simulink model "pfb_fft"  (Simulink 7.0)
settings: Solver=FixedStepDiscrete  SolverMode=SingleTasking  StartTime=0.0  StopTime=2500  RelTol=1e-3
libraries: xbsIndex_r4 x1144
(part 12 of 20)

== system pfb_fft/r4_dit_fft/r4_dit_stage_5/r4_butterfly/butterfly2 ==
  a : Inport  OutDataType=sfix(16)  OutScaling=2^0
  b : Inport  Port=2  OutDataType=sfix(16)  OutScaling=2^0
  sync_in : Inport  Port=3  OutDataType=sfix(16)  OutScaling=2^0
  Delay : xbsIndex_r4/Delay  en=off  latency=1  dbl_ovrd=off  reg_retiming=off  block_type=delay
      settings: xl_area=[1 1 0 0 0 0 0]
  add_im : xbsIndex_r4/AddSub  mode=Addition  use_carryin=off  use_carryout=off  en=off  latency=1  precision=Full  arith_type=Unsigned  n_bits=8  bin_pt=2  quantization=Truncate  overflow=Wrap  dbl_ovrd=off  use_behavioral_HDL=on  pipelined=on  use_rpm=on  hw_selection=Fabric  block_type=addsub
      settings: xl_area=[10 19 0 19 0 0 0]  block_version=10.1.3
  add_re : xbsIndex_r4/AddSub  mode=Addition  use_carryin=off  use_carryout=off  en=off  latency=1  precision=Full  arith_type=Unsigned  n_bits=8  bin_pt=2  quantization=Truncate  overflow=Wrap  dbl_ovrd=off  use_behavioral_HDL=on  pipelined=on  use_rpm=on  hw_selection=Fabric  block_type=addsub
      settings: xl_area=[10 19 0 19 0 0 0]  block_version=10.1.3
  c_to_ri : Subsystem  mask(Complex to Real-Imag){n_bits=18, bin_pt=0}
      mask prompts: n_bits "Bit Width"; bin_pt "Binary Point"
      mask help: Outputs real and imaginary components of a complex input.
      settings: AttributesFormatString=18_0 r/i
      mask Help:
      | <pre>
      | Description::
      | 
      | Outputs real and imaginary components of a complex input.
      | Useful for simplifying interconnects.
      | See also: Real-Imag to Complex (ri_to_c)
      | 
      | Mask Parameters::
      | 
      | Bit Width (n_bits): Specifies the width of the real/imaginary components.
      | Assumed equal for both components.
      | 
      | Binary Point (bin_pt): Specifies the binary point location in the real/imaginary components.
      | Assumed equal for both components.
      | </pre>
  c_to_ri1 : Subsystem  mask(Complex to Real-Imag){n_bits=18, bin_pt=0}
      mask prompts: n_bits "Bit Width"; bin_pt "Binary Point"
      mask help: Outputs real and imaginary components of a complex input.
      settings: AttributesFormatString=18_0 r/i
      mask Help:
      | <pre>
      | Description::
      | 
      | Outputs real and imaginary components of a complex input.
      | Useful for simplifying interconnects.
      | See also: Real-Imag to Complex (ri_to_c)
      | 
      | Mask Parameters::
      | 
      | Bit Width (n_bits): Specifies the width of the real/imaginary components.
      | Assumed equal for both components.
      | 
      | Binary Point (bin_pt): Specifies the binary point location in the real/imaginary components.
      | Assumed equal for both components.
      | </pre>
  requant{0..3} (4 alike) : xbsIndex_r4/Convert  arith_type="Signed  (2's comp)"  n_bits=19  bin_pt=0  quantization=Truncate  overflow=Wrap  latency=0  dbl_ovrd=off  pipeline=on  block_type=convert
      settings: xl_area=[0 0 0 0 0 0 0]  block_version=10.1.3
  ri_to_c : Subsystem
      mask Type: Real-Imag to Complex
      mask Description: Concatenates real and imaginary inputs into a complex output.
      mask Help:
      | <pre>
      | Description::
      | 
      | Concatenates a real and imaginary input into a complex output.
      | Useful for simplifying interconnects.
      | See also: Complex to Real-Imag (c_to_ri)
      | 
      | Mask Parameters::
      | 
      | (N/A)
      | </pre>
  ri_to_c1 : Subsystem
      mask Type: Real-Imag to Complex
      mask Description: Concatenates real and imaginary inputs into a complex output.
      mask Help:
      | <pre>
      | Description::
      | 
      | Concatenates a real and imaginary input into a complex output.
      | Useful for simplifying interconnects.
      | See also: Complex to Real-Imag (c_to_ri)
      | 
      | Mask Parameters::
      | 
      | (N/A)
      | </pre>
  shift{0..3} (4 alike) : xbsIndex_r4/Scale  scale_factor=0  dbl_ovrd=off  block_type=scale
      settings: infoedit=Scales input by a power of two by adjusting the binary point position.<P><P>Hardware notes: In hardware this block costs nothing.  block_version=10.1.3
  sub_im : xbsIndex_r4/AddSub  mode=Subtraction  use_carryin=off  use_carryout=off  en=off  latency=1  precision=Full  arith_type=Unsigned  n_bits=8  bin_pt=2  quantization=Truncate  overflow=Wrap  dbl_ovrd=off  use_behavioral_HDL=on  pipelined=on  use_rpm=on  hw_selection=Fabric  block_type=addsub
      settings: xl_area=[10 19 0 19 0 0 0]  block_version=10.1.3
  sub_re : xbsIndex_r4/AddSub  mode=Subtraction  use_carryin=off  use_carryout=off  en=off  latency=1  precision=Full  arith_type=Unsigned  n_bits=8  bin_pt=2  quantization=Truncate  overflow=Wrap  dbl_ovrd=off  use_behavioral_HDL=on  pipelined=on  use_rpm=on  hw_selection=Fabric  block_type=addsub
      settings: xl_area=[10 19 0 19 0 0 0]  block_version=10.1.3
  a+b : Outport  OutDataType=sfix(16)  OutScaling=2^0
  a-b : Outport  Port=2  OutDataType=sfix(16)  OutScaling=2^0
  sync_out : Outport  Port=3  OutDataType=sfix(16)  OutScaling=2^0
  wires:
  shift3/1 -> requant3/1
  sub_im/1 -> shift3/1
  shift2/1 -> requant2/1
  sub_re/1 -> shift2/1
  shift1/1 -> requant1/1
  shift0/1 -> requant0/1
  requant3/1 -> ri_to_c1/2(im)
  requant2/1 -> ri_to_c1/1(re)
  requant1/1 -> ri_to_c/2(im)
  requant0/1 -> ri_to_c/1(re)
  Delay/1 -> sync_out/1
  sync_in/1 -> Delay/1
  ri_to_c1/1(c) -> a-b/1
  ri_to_c/1(c) -> a+b/1
  add_im/1 -> shift1/1
  add_re/1 -> shift0/1
  a/1 -> c_to_ri/1(c)
  c_to_ri/2(im) -> sub_im/1, add_im/1
  c_to_ri/1(re) -> sub_re/1, add_re/1
  c_to_ri1/2(im) -> add_im/2, sub_im/2
  c_to_ri1/1(re) -> add_re/2, sub_re/2
  b/1 -> c_to_ri1/1(c)

== system pfb_fft/r4_dit_fft/r4_dit_stage_5/r4_butterfly/butterfly3j ==
  a : Inport  OutDataType=sfix(16)  OutScaling=2^0
  b : Inport  Port=2  OutDataType=sfix(16)  OutScaling=2^0
  sync_in : Inport  Port=3  OutDataType=sfix(16)  OutScaling=2^0
  Delay : xbsIndex_r4/Delay  en=off  latency=1  dbl_ovrd=off  reg_retiming=off  block_type=delay
      settings: xl_area=[1 1 0 0 0 0 0]
  add_im : xbsIndex_r4/AddSub  mode=Subtraction  use_carryin=off  use_carryout=off  en=off  latency=1  precision=Full  arith_type=Unsigned  n_bits=8  bin_pt=2  quantization=Truncate  overflow=Wrap  dbl_ovrd=off  use_behavioral_HDL=on  pipelined=on  use_rpm=on  hw_selection=Fabric  block_type=addsub
      settings: xl_area=[10 19 0 19 0 0 0]  block_version=10.1.3
  add_re : xbsIndex_r4/AddSub  mode=Addition  use_carryin=off  use_carryout=off  en=off  latency=1  precision=Full  arith_type=Unsigned  n_bits=8  bin_pt=2  quantization=Truncate  overflow=Wrap  dbl_ovrd=off  use_behavioral_HDL=on  pipelined=on  use_rpm=on  hw_selection=Fabric  block_type=addsub
      settings: xl_area=[10 19 0 19 0 0 0]  block_version=10.1.3
  c_to_ri : Subsystem  mask(Complex to Real-Imag){n_bits=18, bin_pt=0}
      mask prompts: n_bits "Bit Width"; bin_pt "Binary Point"
      mask help: Outputs real and imaginary components of a complex input.
      settings: AttributesFormatString=18_0 r/i
      mask Help:
      | <pre>
      | Description::
      | 
      | Outputs real and imaginary components of a complex input.
      | Useful for simplifying interconnects.
      | See also: Real-Imag to Complex (ri_to_c)
      | 
      | Mask Parameters::
      | 
      | Bit Width (n_bits): Specifies the width of the real/imaginary components.
      | Assumed equal for both components.
      | 
      | Binary Point (bin_pt): Specifies the binary point location in the real/imaginary components.
      | Assumed equal for both components.
      | </pre>
  c_to_ri1 : Subsystem  mask(Complex to Real-Imag){n_bits=18, bin_pt=0}
      mask prompts: n_bits "Bit Width"; bin_pt "Binary Point"
      mask help: Outputs real and imaginary components of a complex input.
      settings: AttributesFormatString=18_0 r/i
      mask Help:
      | <pre>
      | Description::
      | 
      | Outputs real and imaginary components of a complex input.
      | Useful for simplifying interconnects.
      | See also: Real-Imag to Complex (ri_to_c)
      | 
      | Mask Parameters::
      | 
      | Bit Width (n_bits): Specifies the width of the real/imaginary components.
      | Assumed equal for both components.
      | 
      | Binary Point (bin_pt): Specifies the binary point location in the real/imaginary components.
      | Assumed equal for both components.
      | </pre>
  requant{0..3} (4 alike) : xbsIndex_r4/Convert  arith_type="Signed  (2's comp)"  n_bits=19  bin_pt=0  quantization=Truncate  overflow=Wrap  latency=0  dbl_ovrd=off  pipeline=on  block_type=convert
      settings: xl_area=[0 0 0 0 0 0 0]  block_version=10.1.3
  ri_to_c : Subsystem
      mask Type: Real-Imag to Complex
      mask Description: Concatenates real and imaginary inputs into a complex output.
      mask Help:
      | <pre>
      | Description::
      | 
      | Concatenates a real and imaginary input into a complex output.
      | Useful for simplifying interconnects.
      | See also: Complex to Real-Imag (c_to_ri)
      | 
      | Mask Parameters::
      | 
      | (N/A)
      | </pre>
  ri_to_c1 : Subsystem
      mask Type: Real-Imag to Complex
      mask Description: Concatenates real and imaginary inputs into a complex output.
      mask Help:
      | <pre>
      | Description::
      | 
      | Concatenates a real and imaginary input into a complex output.
      | Useful for simplifying interconnects.
      | See also: Complex to Real-Imag (c_to_ri)
      | 
      | Mask Parameters::
      | 
      | (N/A)
      | </pre>
  shift{0..3} (4 alike) : xbsIndex_r4/Scale  scale_factor=0  dbl_ovrd=off  block_type=scale
      settings: infoedit=Scales input by a power of two by adjusting the binary point position.<P><P>Hardware notes: In hardware this block costs nothing.  block_version=10.1.3
  sub_im : xbsIndex_r4/AddSub  mode=Addition  use_carryin=off  use_carryout=off  en=off  latency=1  precision=Full  arith_type=Unsigned  n_bits=8  bin_pt=2  quantization=Truncate  overflow=Wrap  dbl_ovrd=off  use_behavioral_HDL=on  pipelined=on  use_rpm=on  hw_selection=Fabric  block_type=addsub
      settings: xl_area=[10 19 0 19 0 0 0]  block_version=10.1.3
  sub_re : xbsIndex_r4/AddSub  mode=Subtraction  use_carryin=off  use_carryout=off  en=off  latency=1  precision=Full  arith_type=Unsigned  n_bits=8  bin_pt=2  quantization=Truncate  overflow=Wrap  dbl_ovrd=off  use_behavioral_HDL=on  pipelined=on  use_rpm=on  hw_selection=Fabric  block_type=addsub
      settings: xl_area=[10 19 0 19 0 0 0]  block_version=10.1.3
  a+b : Outport  OutDataType=sfix(16)  OutScaling=2^0
  a-b : Outport  Port=2  OutDataType=sfix(16)  OutScaling=2^0
  sync_out : Outport  Port=3  OutDataType=sfix(16)  OutScaling=2^0
  wires:
  requant3/1 -> ri_to_c1/2(im)
  requant2/1 -> ri_to_c1/1(re)
  requant1/1 -> ri_to_c/2(im)
  requant0/1 -> ri_to_c/1(re)
  shift3/1 -> requant3/1
  shift2/1 -> requant2/1
  shift1/1 -> requant1/1
  shift0/1 -> requant0/1
  sub_im/1 -> shift3/1
  sub_re/1 -> shift2/1
  b/1 -> c_to_ri1/1(c)
  c_to_ri1/1(re) -> add_im/2, sub_im/2
  c_to_ri1/2(im) -> add_re/2, sub_re/2
  c_to_ri/1(re) -> sub_re/1, add_re/1
  c_to_ri/2(im) -> sub_im/1, add_im/1
  a/1 -> c_to_ri/1(c)
  add_re/1 -> shift0/1
  add_im/1 -> shift1/1
  ri_to_c/1(c) -> a+b/1
  ri_to_c1/1(c) -> a-b/1
  sync_in/1 -> Delay/1
  Delay/1 -> sync_out/1

== system pfb_fft/r4_dit_fft/r4_dit_stage_5/r4_twiddle/cmpy1 ==
  a_in : Inport  OutDataType=sfix(16)  OutScaling=2^0
  b : Inport  Port=2  OutDataType=sfix(16)  OutScaling=2^0
  w : Inport  Port=3  OutDataType=sfix(16)  OutScaling=2^0
  sync_in : Inport  Port=4  OutDataType=sfix(16)  OutScaling=2^0
  Delay : xbsIndex_r4/Delay  en=off  latency=8  dbl_ovrd=off  reg_retiming=off  block_type=delay
      settings: xl_area=[1 1 0 1 0 0 0]
  Delay1 : xbsIndex_r4/Delay  en=off  latency=8  dbl_ovrd=off  reg_retiming=off  block_type=delay
      settings: xl_area=[17 34 0 34 0 0 0]
  br_add_bi : xbsIndex_r4/AddSub  mode=Addition  use_carryin=off  use_carryout=off  en=off  latency=1  precision=Full  arith_type=Unsigned  n_bits=8  bin_pt=2  quantization=Truncate  overflow=Wrap  dbl_ovrd=off  use_behavioral_HDL=on  pipelined=on  use_rpm=on  hw_selection=Fabric  block_type=addsub
      settings: xl_area=[9 18 0 18 0 0 0]  block_version=10.1.3
  c_to_ri : Subsystem  mask(Complex to Real-Imag){n_bits=17, bin_pt=16}
      mask prompts: n_bits "Bit Width"; bin_pt "Binary Point"
      mask help: Outputs real and imaginary components of a complex input.
      settings: AttributesFormatString=17_16 r/i
      mask Help:
      | <pre>
      | Description::
      | 
      | Outputs real and imaginary components of a complex input.
      | Useful for simplifying interconnects.
      | See also: Real-Imag to Complex (ri_to_c)
      | 
      | Mask Parameters::
      | 
      | Bit Width (n_bits): Specifies the width of the real/imaginary components.
      | Assumed equal for both components.
      | 
      | Binary Point (bin_pt): Specifies the binary point location in the real/imaginary components.
      | Assumed equal for both components.
      | </pre>
  c_to_ri1 : Subsystem  mask(Complex to Real-Imag){n_bits=9, bin_pt=7}
      mask prompts: n_bits "Bit Width"; bin_pt "Binary Point"
      mask help: Outputs real and imaginary components of a complex input.
      settings: AttributesFormatString=9_7 r/i
      mask Help:
      | <pre>
      | Description::
      | 
      | Outputs real and imaginary components of a complex input.
      | Useful for simplifying interconnects.
      | See also: Real-Imag to Complex (ri_to_c)
      | 
      | Mask Parameters::
      | 
      | Bit Width (n_bits): Specifies the width of the real/imaginary components.
      | Assumed equal for both components.
      | 
      | Binary Point (bin_pt): Specifies the binary point location in the real/imaginary components.
      | Assumed equal for both components.
      | </pre>
  convert_im : xbsIndex_r4/Convert  arith_type="Signed  (2's comp)"  n_bits=17  bin_pt=16  quantization="Round  (unbiased: Even Values)"  overflow=Wrap  latency=3  dbl_ovrd=off  pipeline=on  block_type=convert
      settings: xl_area=[21 17 0 37 0 0 0]  block_version=10.1.3
  convert_re : xbsIndex_r4/Convert  arith_type="Signed  (2's comp)"  n_bits=17  bin_pt=16  quantization="Round  (unbiased: Even Values)"  overflow=Wrap  latency=3  dbl_ovrd=off  pipeline=on  block_type=convert
      settings: xl_area=[21 17 0 37 0 0 0]  block_version=10.1.3
  imim : xbsIndex_r4/Mult  precision=User Defined  arith_type="Signed  (2's comp)"  n_bits=24  bin_pt=23  quantization=Truncate  overflow=Wrap  en=off  latency=3  dbl_ovrd=off  use_behavioral_HDL=off  use_embedded=on  opt=Speed  optimum_pipeline=off  pipeline=on  use_rpm=on  placement_style=Rectangular shape  block_type=mult
      settings: infoedit=Hardware notes: To use the internal pipeline stage of the dedicated multiplier you must select 'Pipeline for maximum performance'.  xl_area=[25 50 0 24 0 1 0]  block_version=10.1.3
  rere : xbsIndex_r4/Mult  precision=User Defined  arith_type="Signed  (2's comp)"  n_bits=24  bin_pt=23  quantization=Truncate  overflow=Wrap  en=off  latency=3  dbl_ovrd=off  use_behavioral_HDL=off  use_embedded=on  opt=Speed  optimum_pipeline=off  pipeline=on  use_rpm=on  placement_style=Rectangular shape  block_type=mult
      settings: infoedit=Hardware notes: To use the internal pipeline stage of the dedicated multiplier you must select 'Pipeline for maximum performance'.  xl_area=[25 50 0 24 0 1 0]  block_version=10.1.3
  ri_to_c : Subsystem
      mask Type: Real-Imag to Complex
      mask Description: Concatenates real and imaginary inputs into a complex output.
      mask Help:
      | <pre>
      | Description::
      | 
      | Concatenates a real and imaginary input into a complex output.
      | Useful for simplifying interconnects.
      | See also: Complex to Real-Imag (c_to_ri)
      | 
      | Mask Parameters::
      | 
      | (N/A)
      | </pre>
  rr_add_ii : xbsIndex_r4/AddSub  mode=Addition  use_carryin=off  use_carryout=off  en=off  latency=1  precision=User Defined  arith_type="Signed  (2's comp)"  n_bits=24  bin_pt=23  quantization=Truncate  overflow=Wrap  dbl_ovrd=off  use_behavioral_HDL=on  pipelined=on  use_rpm=on  hw_selection=Fabric  block_type=addsub
      settings: xl_area=[12 24 0 24 0 0 0]  block_version=10.1.3
  rr_sub_ii : xbsIndex_r4/AddSub  mode=Subtraction  use_carryin=off  use_carryout=off  en=off  latency=2  precision=User Defined  arith_type="Signed  (2's comp)"  n_bits=24  bin_pt=23  quantization=Truncate  overflow=Wrap  dbl_ovrd=off  use_behavioral_HDL=on  pipelined=on  use_rpm=on  hw_selection=Fabric  block_type=addsub
      settings: xl_area=[24 48 0 24 0 0 0]  block_version=10.1.3
  ss_sub_rrii : xbsIndex_r4/AddSub  mode=Subtraction  use_carryin=off  use_carryout=off  en=off  latency=1  precision=User Defined  arith_type="Signed  (2's comp)"  n_bits=24  bin_pt=23  quantization=Truncate  overflow=Wrap  dbl_ovrd=off  use_behavioral_HDL=on  pipelined=on  use_rpm=on  hw_selection=Fabric  block_type=addsub
      settings: xl_area=[12 24 0 24 0 0 0]  block_version=10.1.3
  sumsum : xbsIndex_r4/Mult  precision=User Defined  arith_type="Signed  (2's comp)"  n_bits=24  bin_pt=23  quantization=Truncate  overflow=Wrap  en=off  latency=3  dbl_ovrd=off  use_behavioral_HDL=off  use_embedded=on  opt=Speed  optimum_pipeline=off  pipeline=on  use_rpm=on  placement_style=Rectangular shape  block_type=mult
      settings: infoedit=Hardware notes: To use the internal pipeline stage of the dedicated multiplier you must select 'Pipeline for maximum performance'.  xl_area=[26 52 0 24 0 1 0]  block_version=10.1.3
  wr_add_wi : xbsIndex_r4/AddSub  mode=Addition  use_carryin=off  use_carryout=off  en=off  latency=1  precision=Full  arith_type=Unsigned  n_bits=8  bin_pt=2  quantization=Truncate  overflow=Wrap  dbl_ovrd=off  use_behavioral_HDL=on  pipelined=on  use_rpm=on  hw_selection=Fabric  block_type=addsub
      settings: xl_area=[5 10 0 10 0 0 0]  block_version=10.1.3
  a_out : Outport  OutDataType=sfix(16)  OutScaling=2^0
  bw : Outport  Port=2  OutDataType=sfix(16)  OutScaling=2^0
  sync_out : Outport  Port=3  OutDataType=sfix(16)  OutScaling=2^0
  wires:
  ss_sub_rrii/1 -> convert_im/1
  rr_sub_ii/1 -> convert_re/1
  rr_add_ii/1 -> ss_sub_rrii/2
  b/1 -> c_to_ri/1(c)
  w/1 -> c_to_ri1/1(c)
  rere/1 -> rr_add_ii/2, rr_sub_ii/1
  imim/1 -> rr_sub_ii/2, rr_add_ii/1
  br_add_bi/1 -> sumsum/1
  wr_add_wi/1 -> sumsum/2
  ri_to_c/1(c) -> bw/1
  sumsum/1 -> ss_sub_rrii/1
  sync_in/1 -> Delay/1
  Delay/1 -> sync_out/1
  c_to_ri/1(re) -> br_add_bi/1, rere/1
  c_to_ri1/2(im) -> imim/2, wr_add_wi/2
  c_to_ri1/1(re) -> rere/2, wr_add_wi/1
  c_to_ri/2(im) -> br_add_bi/2, imim/1
  a_in/1 -> Delay1/1
  Delay1/1 -> a_out/1
  convert_re/1 -> ri_to_c/1(re)
  convert_im/1 -> ri_to_c/2(im)

== system pfb_fft/r4_dit_fft/r4_dit_stage_5/r4_twiddle/cmpy2 ==
  a_in : Inport  OutDataType=sfix(16)  OutScaling=2^0
  b : Inport  Port=2  OutDataType=sfix(16)  OutScaling=2^0
  w : Inport  Port=3  OutDataType=sfix(16)  OutScaling=2^0
  sync_in : Inport  Port=4  OutDataType=sfix(16)  OutScaling=2^0
  Delay : xbsIndex_r4/Delay  en=off  latency=8  dbl_ovrd=off  reg_retiming=off  block_type=delay
      settings: xl_area=[1 1 0 1 0 0 0]
  Delay1 : xbsIndex_r4/Delay  en=off  latency=8  dbl_ovrd=off  reg_retiming=off  block_type=delay
      settings: xl_area=[1 1 0 1 0 0 0]
  br_add_bi : xbsIndex_r4/AddSub  mode=Addition  use_carryin=off  use_carryout=off  en=off  latency=1  precision=Full  arith_type=Unsigned  n_bits=8  bin_pt=2  quantization=Truncate  overflow=Wrap  dbl_ovrd=off  use_behavioral_HDL=on  pipelined=on  use_rpm=on  hw_selection=Fabric  block_type=addsub
      settings: xl_area=[9 18 0 18 0 0 0]  block_version=10.1.3
  c_to_ri : Subsystem  mask(Complex to Real-Imag){n_bits=17, bin_pt=16}
      mask prompts: n_bits "Bit Width"; bin_pt "Binary Point"
      mask help: Outputs real and imaginary components of a complex input.
      settings: AttributesFormatString=17_16 r/i
      mask Help:
      | <pre>
      | Description::
      | 
      | Outputs real and imaginary components of a complex input.
      | Useful for simplifying interconnects.
      | See also: Real-Imag to Complex (ri_to_c)
      | 
      | Mask Parameters::
      | 
      | Bit Width (n_bits): Specifies the width of the real/imaginary components.
      | Assumed equal for both components.
      | 
      | Binary Point (bin_pt): Specifies the binary point location in the real/imaginary components.
      | Assumed equal for both components.
      | </pre>
  c_to_ri1 : Subsystem  mask(Complex to Real-Imag){n_bits=9, bin_pt=7}
      mask prompts: n_bits "Bit Width"; bin_pt "Binary Point"
      mask help: Outputs real and imaginary components of a complex input.
      settings: AttributesFormatString=9_7 r/i
      mask Help:
      | <pre>
      | Description::
      | 
      | Outputs real and imaginary components of a complex input.
      | Useful for simplifying interconnects.
      | See also: Real-Imag to Complex (ri_to_c)
      | 
      | Mask Parameters::
      | 
      | Bit Width (n_bits): Specifies the width of the real/imaginary components.
      | Assumed equal for both components.
      | 
      | Binary Point (bin_pt): Specifies the binary point location in the real/imaginary components.
      | Assumed equal for both components.
      | </pre>
  convert_im : xbsIndex_r4/Convert  arith_type="Signed  (2's comp)"  n_bits=17  bin_pt=16  quantization="Round  (unbiased: Even Values)"  overflow=Wrap  latency=3  dbl_ovrd=off  pipeline=on  block_type=convert
      settings: xl_area=[21 17 0 37 0 0 0]  block_version=10.1.3
  convert_re : xbsIndex_r4/Convert  arith_type="Signed  (2's comp)"  n_bits=17  bin_pt=16  quantization="Round  (unbiased: Even Values)"  overflow=Wrap  latency=3  dbl_ovrd=off  pipeline=on  block_type=convert
      settings: xl_area=[21 17 0 37 0 0 0]  block_version=10.1.3
  imim : xbsIndex_r4/Mult  precision=User Defined  arith_type="Signed  (2's comp)"  n_bits=24  bin_pt=23  quantization=Truncate  overflow=Wrap  en=off  latency=3  dbl_ovrd=off  use_behavioral_HDL=off  use_embedded=on  opt=Speed  optimum_pipeline=off  pipeline=on  use_rpm=on  placement_style=Rectangular shape  block_type=mult
      settings: infoedit=Hardware notes: To use the internal pipeline stage of the dedicated multiplier you must select 'Pipeline for maximum performance'.  xl_area=[25 50 0 24 0 1 0]  block_version=10.1.3
  rere : xbsIndex_r4/Mult  precision=User Defined  arith_type="Signed  (2's comp)"  n_bits=24  bin_pt=23  quantization=Truncate  overflow=Wrap  en=off  latency=3  dbl_ovrd=off  use_behavioral_HDL=off  use_embedded=on  opt=Speed  optimum_pipeline=off  pipeline=on  use_rpm=on  placement_style=Rectangular shape  block_type=mult
      settings: infoedit=Hardware notes: To use the internal pipeline stage of the dedicated multiplier you must select 'Pipeline for maximum performance'.  xl_area=[25 50 0 24 0 1 0]  block_version=10.1.3
  ri_to_c : Subsystem
      mask Type: Real-Imag to Complex
      mask Description: Concatenates real and imaginary inputs into a complex output.
      mask Help:
      | <pre>
      | Description::
      | 
      | Concatenates a real and imaginary input into a complex output.
      | Useful for simplifying interconnects.
      | See also: Complex to Real-Imag (c_to_ri)
      | 
      | Mask Parameters::
      | 
      | (N/A)
      | </pre>
  rr_add_ii : xbsIndex_r4/AddSub  mode=Addition  use_carryin=off  use_carryout=off  en=off  latency=1  precision=User Defined  arith_type="Signed  (2's comp)"  n_bits=24  bin_pt=23  quantization=Truncate  overflow=Wrap  dbl_ovrd=off  use_behavioral_HDL=on  pipelined=on  use_rpm=on  hw_selection=Fabric  block_type=addsub
      settings: xl_area=[12 24 0 24 0 0 0]  block_version=10.1.3
  rr_sub_ii : xbsIndex_r4/AddSub  mode=Subtraction  use_carryin=off  use_carryout=off  en=off  latency=2  precision=User Defined  arith_type="Signed  (2's comp)"  n_bits=24  bin_pt=23  quantization=Truncate  overflow=Wrap  dbl_ovrd=off  use_behavioral_HDL=on  pipelined=on  use_rpm=on  hw_selection=Fabric  block_type=addsub
      settings: xl_area=[24 48 0 24 0 0 0]  block_version=10.1.3
  ss_sub_rrii : xbsIndex_r4/AddSub  mode=Subtraction  use_carryin=off  use_carryout=off  en=off  latency=1  precision=User Defined  arith_type="Signed  (2's comp)"  n_bits=24  bin_pt=23  quantization=Truncate  overflow=Wrap  dbl_ovrd=off  use_behavioral_HDL=on  pipelined=on  use_rpm=on  hw_selection=Fabric  block_type=addsub
      settings: xl_area=[12 24 0 24 0 0 0]  block_version=10.1.3
  sumsum : xbsIndex_r4/Mult  precision=User Defined  arith_type="Signed  (2's comp)"  n_bits=24  bin_pt=23  quantization=Truncate  overflow=Wrap  en=off  latency=3  dbl_ovrd=off  use_behavioral_HDL=off  use_embedded=on  opt=Speed  optimum_pipeline=off  pipeline=on  use_rpm=on  placement_style=Rectangular shape  block_type=mult
      settings: infoedit=Hardware notes: To use the internal pipeline stage of the dedicated multiplier you must select 'Pipeline for maximum performance'.  xl_area=[26 52 0 24 0 1 0]  block_version=10.1.3
  wr_add_wi : xbsIndex_r4/AddSub  mode=Addition  use_carryin=off  use_carryout=off  en=off  latency=1  precision=Full  arith_type=Unsigned  n_bits=8  bin_pt=2  quantization=Truncate  overflow=Wrap  dbl_ovrd=off  use_behavioral_HDL=on  pipelined=on  use_rpm=on  hw_selection=Fabric  block_type=addsub
      settings: xl_area=[5 10 0 10 0 0 0]  block_version=10.1.3
  a_out : Outport  OutDataType=sfix(16)  OutScaling=2^0
  bw : Outport  Port=2  OutDataType=sfix(16)  OutScaling=2^0
  sync_out : Outport  Port=3  OutDataType=sfix(16)  OutScaling=2^0
  wires:
  ss_sub_rrii/1 -> convert_im/1
  rr_sub_ii/1 -> convert_re/1
  rr_add_ii/1 -> ss_sub_rrii/2
  b/1 -> c_to_ri/1(c)
  w/1 -> c_to_ri1/1(c)
  rere/1 -> rr_add_ii/2, rr_sub_ii/1
  imim/1 -> rr_sub_ii/2, rr_add_ii/1
  br_add_bi/1 -> sumsum/1
  wr_add_wi/1 -> sumsum/2
  ri_to_c/1(c) -> bw/1
  sumsum/1 -> ss_sub_rrii/1
  sync_in/1 -> Delay/1
  Delay/1 -> sync_out/1
  c_to_ri/1(re) -> br_add_bi/1, rere/1
  c_to_ri1/2(im) -> imim/2, wr_add_wi/2
  c_to_ri1/1(re) -> rere/2, wr_add_wi/1
  c_to_ri/2(im) -> br_add_bi/2, imim/1
  a_in/1 -> Delay1/1
  Delay1/1 -> a_out/1
  convert_re/1 -> ri_to_c/1(re)
  convert_im/1 -> ri_to_c/2(im)

== system pfb_fft/r4_dit_fft/r4_dit_stage_5/r4_twiddle/cmpy3 ==
  a_in : Inport  OutDataType=sfix(16)  OutScaling=2^0
  b : Inport  Port=2  OutDataType=sfix(16)  OutScaling=2^0
  w : Inport  Port=3  OutDataType=sfix(16)  OutScaling=2^0
  sync_in : Inport  Port=4  OutDataType=sfix(16)  OutScaling=2^0
  Delay : xbsIndex_r4/Delay  en=off  latency=8  dbl_ovrd=off  reg_retiming=off  block_type=delay
      settings: xl_area=[1 1 0 1 0 0 0]
  Delay1 : xbsIndex_r4/Delay  en=off  latency=8  dbl_ovrd=off  reg_retiming=off  block_type=delay
      settings: xl_area=[1 1 0 1 0 0 0]
  br_add_bi : xbsIndex_r4/AddSub  mode=Addition  use_carryin=off  use_carryout=off  en=off  latency=1  precision=Full  arith_type=Unsigned  n_bits=8  bin_pt=2  quantization=Truncate  overflow=Wrap  dbl_ovrd=off  use_behavioral_HDL=on  pipelined=on  use_rpm=on  hw_selection=Fabric  block_type=addsub
      settings: xl_area=[9 18 0 18 0 0 0]  block_version=10.1.3
  c_to_ri : Subsystem  mask(Complex to Real-Imag){n_bits=17, bin_pt=16}
      mask prompts: n_bits "Bit Width"; bin_pt "Binary Point"
      mask help: Outputs real and imaginary components of a complex input.
      settings: AttributesFormatString=17_16 r/i
      mask Help:
      | <pre>
      | Description::
      | 
      | Outputs real and imaginary components of a complex input.
      | Useful for simplifying interconnects.
      | See also: Real-Imag to Complex (ri_to_c)
      | 
      | Mask Parameters::
      | 
      | Bit Width (n_bits): Specifies the width of the real/imaginary components.
      | Assumed equal for both components.
      | 
      | Binary Point (bin_pt): Specifies the binary point location in the real/imaginary components.
      | Assumed equal for both components.
      | </pre>
  c_to_ri1 : Subsystem  mask(Complex to Real-Imag){n_bits=9, bin_pt=7}
      mask prompts: n_bits "Bit Width"; bin_pt "Binary Point"
      mask help: Outputs real and imaginary components of a complex input.
      settings: AttributesFormatString=9_7 r/i
      mask Help:
      | <pre>
      | Description::
      | 
      | Outputs real and imaginary components of a complex input.
      | Useful for simplifying interconnects.
      | See also: Real-Imag to Complex (ri_to_c)
      | 
      | Mask Parameters::
      | 
      | Bit Width (n_bits): Specifies the width of the real/imaginary components.
      | Assumed equal for both components.
      | 
      | Binary Point (bin_pt): Specifies the binary point location in the real/imaginary components.
      | Assumed equal for both components.
      | </pre>
  convert_im : xbsIndex_r4/Convert  arith_type="Signed  (2's comp)"  n_bits=17  bin_pt=16  quantization="Round  (unbiased: Even Values)"  overflow=Wrap  latency=3  dbl_ovrd=off  pipeline=on  block_type=convert
      settings: xl_area=[21 17 0 37 0 0 0]  block_version=10.1.3
  convert_re : xbsIndex_r4/Convert  arith_type="Signed  (2's comp)"  n_bits=17  bin_pt=16  quantization="Round  (unbiased: Even Values)"  overflow=Wrap  latency=3  dbl_ovrd=off  pipeline=on  block_type=convert
      settings: xl_area=[21 17 0 37 0 0 0]  block_version=10.1.3
  imim : xbsIndex_r4/Mult  precision=User Defined  arith_type="Signed  (2's comp)"  n_bits=24  bin_pt=23  quantization=Truncate  overflow=Wrap  en=off  latency=3  dbl_ovrd=off  use_behavioral_HDL=off  use_embedded=on  opt=Speed  optimum_pipeline=off  pipeline=on  use_rpm=on  placement_style=Rectangular shape  block_type=mult
      settings: infoedit=Hardware notes: To use the internal pipeline stage of the dedicated multiplier you must select 'Pipeline for maximum performance'.  xl_area=[25 50 0 24 0 1 0]  block_version=10.1.3
  rere : xbsIndex_r4/Mult  precision=User Defined  arith_type="Signed  (2's comp)"  n_bits=24  bin_pt=23  quantization=Truncate  overflow=Wrap  en=off  latency=3  dbl_ovrd=off  use_behavioral_HDL=off  use_embedded=on  opt=Speed  optimum_pipeline=off  pipeline=on  use_rpm=on  placement_style=Rectangular shape  block_type=mult
      settings: infoedit=Hardware notes: To use the internal pipeline stage of the dedicated multiplier you must select 'Pipeline for maximum performance'.  xl_area=[25 50 0 24 0 1 0]  block_version=10.1.3
  ri_to_c : Subsystem
      mask Type: Real-Imag to Complex
      mask Description: Concatenates real and imaginary inputs into a complex output.
      mask Help:
      | <pre>
      | Description::
      | 
      | Concatenates a real and imaginary input into a complex output.
      | Useful for simplifying interconnects.
      | See also: Complex to Real-Imag (c_to_ri)
      | 
      | Mask Parameters::
      | 
      | (N/A)
      | </pre>
  rr_add_ii : xbsIndex_r4/AddSub  mode=Addition  use_carryin=off  use_carryout=off  en=off  latency=1  precision=User Defined  arith_type="Signed  (2's comp)"  n_bits=24  bin_pt=23  quantization=Truncate  overflow=Wrap  dbl_ovrd=off  use_behavioral_HDL=on  pipelined=on  use_rpm=on  hw_selection=Fabric  block_type=addsub
      settings: xl_area=[12 24 0 24 0 0 0]  block_version=10.1.3
  rr_sub_ii : xbsIndex_r4/AddSub  mode=Subtraction  use_carryin=off  use_carryout=off  en=off  latency=2  precision=User Defined  arith_type="Signed  (2's comp)"  n_bits=24  bin_pt=23  quantization=Truncate  overflow=Wrap  dbl_ovrd=off  use_behavioral_HDL=on  pipelined=on  use_rpm=on  hw_selection=Fabric  block_type=addsub
      settings: xl_area=[24 48 0 24 0 0 0]  block_version=10.1.3
  ss_sub_rrii : xbsIndex_r4/AddSub  mode=Subtraction  use_carryin=off  use_carryout=off  en=off  latency=1  precision=User Defined  arith_type="Signed  (2's comp)"  n_bits=24  bin_pt=23  quantization=Truncate  overflow=Wrap  dbl_ovrd=off  use_behavioral_HDL=on  pipelined=on  use_rpm=on  hw_selection=Fabric  block_type=addsub
      settings: xl_area=[12 24 0 24 0 0 0]  block_version=10.1.3
  sumsum : xbsIndex_r4/Mult  precision=User Defined  arith_type="Signed  (2's comp)"  n_bits=24  bin_pt=23  quantization=Truncate  overflow=Wrap  en=off  latency=3  dbl_ovrd=off  use_behavioral_HDL=off  use_embedded=on  opt=Speed  optimum_pipeline=off  pipeline=on  use_rpm=on  placement_style=Rectangular shape  block_type=mult
      settings: infoedit=Hardware notes: To use the internal pipeline stage of the dedicated multiplier you must select 'Pipeline for maximum performance'.  xl_area=[26 52 0 24 0 1 0]  block_version=10.1.3
  wr_add_wi : xbsIndex_r4/AddSub  mode=Addition  use_carryin=off  use_carryout=off  en=off  latency=1  precision=Full  arith_type=Unsigned  n_bits=8  bin_pt=2  quantization=Truncate  overflow=Wrap  dbl_ovrd=off  use_behavioral_HDL=on  pipelined=on  use_rpm=on  hw_selection=Fabric  block_type=addsub
      settings: xl_area=[5 10 0 10 0 0 0]  block_version=10.1.3
  a_out : Outport  OutDataType=sfix(16)  OutScaling=2^0
  bw : Outport  Port=2  OutDataType=sfix(16)  OutScaling=2^0
  sync_out : Outport  Port=3  OutDataType=sfix(16)  OutScaling=2^0
  wires:
  ss_sub_rrii/1 -> convert_im/1
  rr_sub_ii/1 -> convert_re/1
  rr_add_ii/1 -> ss_sub_rrii/2
  b/1 -> c_to_ri/1(c)
  w/1 -> c_to_ri1/1(c)
  rere/1 -> rr_add_ii/2, rr_sub_ii/1
  imim/1 -> rr_sub_ii/2, rr_add_ii/1
  br_add_bi/1 -> sumsum/1
  wr_add_wi/1 -> sumsum/2
  ri_to_c/1(c) -> bw/1
  sumsum/1 -> ss_sub_rrii/1
  sync_in/1 -> Delay/1
  Delay/1 -> sync_out/1
  c_to_ri/1(re) -> br_add_bi/1, rere/1
  c_to_ri1/2(im) -> imim/2, wr_add_wi/2
  c_to_ri1/1(re) -> rere/2, wr_add_wi/1
  c_to_ri/2(im) -> br_add_bi/2, imim/1
  a_in/1 -> Delay1/1
  Delay1/1 -> a_out/1
  convert_re/1 -> ri_to_c/1(re)
  convert_im/1 -> ri_to_c/2(im)

== system pfb_fft/r4_dit_fft/r4_dit_stage_5/r4_twiddle/twiddle_gen1 ==
  sync_in : Inport  OutDataType=sfix(16)  OutScaling=2^0
  Counter : xbsIndex_r4/Counter  cnt_type=Free Running  cnt_to=Inf  operation=Up  start_count=0  cnt_by_val=1  arith_type=Unsigned  n_bits=8  bin_pt=0  load_pin=off  rst=on  en=off  explicit_period=off  period=1  dbl_ovrd=off  use_behavioral_HDL=off  use_rpm=on  implementation=Fabric  block_type=counter
      settings: xl_area=[4 8 0 8 0 0 0]
  addr_sel : xbsIndex_r4/Slice  nbits=8  boolean_output=off  mode=Upper Bit Location + Width  bit1=0  base1=MSB of Input  bit0=-1  base0=MSB of Input  dbl_ovrd=off  block_type=slice
      settings: infoedit="Extracts a given range of bits from each input sample and presents it at the output.  The output type is ordinarily unsigned with binary point at zero, but can be Boolean when the slice is one bit wide.<P><P>Hardware notes: In hardware this block costs nothing."  block_version=10.1.3
  mem_c : xbsIndex_r4/ROM  depth=256  initVector=[65536;47013;60879;25482;64999;36758;54713;13186;65523;41885;58308;19334;62939;31119;51119;7041;66042;44449;59849;22407;63969;34194;53172;10113;65517;39321;56766;16260;62421;28556;49066;3456;66045;45475;60364;23945;64484;35220;54198;11650;65520;40859;57281;17797;62936;30094;50092;4992;66039;43423;58822;20870;63454;32657;52145;8577;65002;38295;55740;14723;61394;27019;48040;1920;66046;45988;60878;24969;64485;36245;54712;12162;65522;41372;57794;18821;62937;30606;50606;6016;66040;43936;59336;21895;63967;33169;52658;9089;65004;38808;56253;15747;61907;27532;48553;2944;66043;44962;59851;23432;64482;34707;53685;10626;65519;40346;57280;17284;62422;29069;49579;4480;66037;42398;58821;20358;63452;32144;51632;7553;65001;37270;55226;14211;61392;25994;47527;1408;66047;46501;60878;24969;64486;36245;54712;12674;65523;41885;58307;18821;62938;31119;50606;6529;66041;43937;59337;21895;63968;33682;52659;9601;65004;39321;56254;15748;61908;28044;48553;2944;66044;45475;60363;23432;64483;35219;53686;11138;65520;40347;57280;17284;62423;29581;49580;4992;66038;42911;58822;20358;63453;32144;51633;8065;65001;37783;55739;14211;61393;26507;47527;1408;66046;45988;60365;24457;64485;35732;54199;12162;65521;40860;57794;18309;62937;30094;50093;5504;66039;43424;59335;21383;63967;33169;52146;8577;65003;38296;56252;15235;61907;27531;48040;2432;66043;44962;59850;22920;63970;34195;53172;10626;65518;39834;56767;16772;62422;28557;49067;3968;65524;42398;58308;19846;63452;31631;51119;7041;65000;37270;55226;13699;61392;25994;47014;896]  distributed_mem=Block RAM  rst=off  init_reg=0  en=off  latency=1  arith_type=Unsigned  n_bits=18  bin_pt=0  dbl_ovrd=off  optimize=Area  use_rpm=on  block_type=sprom
      settings: AttributesFormatString=depth = %<depth>\ndist_mem = %<distributed_mem>  xl_area=[0 0 1 0 0 0 0]  block_version=10.1.3
  w : Outport  OutDataType=sfix(16)  OutScaling=2^0
  wires:
  mem_c/1 -> w/1
  addr_sel/1 -> mem_c/1
  Counter/1 -> addr_sel/1
  sync_in/1 -> Counter/1

== system pfb_fft/r4_dit_fft/r4_dit_stage_5/r4_twiddle/twiddle_gen2 ==
  sync_in : Inport  OutDataType=sfix(16)  OutScaling=2^0
  Counter : xbsIndex_r4/Counter  cnt_type=Free Running  cnt_to=Inf  operation=Up  start_count=0  cnt_by_val=1  arith_type=Unsigned  n_bits=8  bin_pt=0  load_pin=off  rst=on  en=off  explicit_period=off  period=1  dbl_ovrd=off  use_behavioral_HDL=off  use_rpm=on  implementation=Fabric  block_type=counter
      settings: xl_area=[4 8 0 8 0 0 0]
  addr_sel : xbsIndex_r4/Slice  nbits=8  boolean_output=off  mode=Upper Bit Location + Width  bit1=0  base1=MSB of Input  bit0=-1  base0=MSB of Input  dbl_ovrd=off  block_type=slice
      settings: infoedit="Extracts a given range of bits from each input sample and presents it at the output.  The output type is ordinarily unsigned with binary point at zero, but can be Boolean when the slice is one bit wide.<P><P>Hardware notes: In hardware this block costs nothing."  block_version=10.1.3
  mem_c : xbsIndex_r4/ROM  depth=256  initVector=[65536;384;47013;215973;60879;237450;25482;202191;64999;249730;36758;208313;54713;226198;13186;198119;65523;255873;41885;211887;58308;231823;19334;200155;62939;243590;31119;204740;51119;221085;7041;197619;66042;259456;44449;213930;59849;234380;22407;200661;63969;246660;34194;206270;53172;223641;10113;197613;65517;252801;39321;209844;56766;228754;16260;199137;62421;240519;28556;203209;49066;218529;3456;197114;66045;260992;45475;214952;60364;235915;23945;201682;64484;248195;35220;207292;54198;224663;11650;198122;65520;254337;40859;210865;57281;230289;17797;199646;62936;242054;30094;204230;50092;219551;4992;197111;66039;257920;43423;212908;58822;232846;20870;200152;63454;245125;32657;205761;52145;222107;8577;197616;65002;251266;38295;208822;55740;227732;14723;198628;61394;238985;27019;202700;48040;217507;1920;197117;66046;261504;45988;215463;60878;236938;24969;201680;64485;248707;36245;207802;54712;225686;12162;198121;65522;255361;41372;211376;57794;230800;18821;199644;62937;242566;30606;204229;50606;220574;6016;197109;66040;258432;43936;213419;59336;233869;21895;200662;63967;245636;33169;205760;52658;222618;9089;197615;65004;252290;38808;209333;56253;228243;15747;198626;61907;239496;27532;203211;48553;218018;2944;197115;66043;259968;44962;214441;59851;235404;23432;201171;64482;247171;34707;206781;53685;224152;10626;198124;65519;253825;40346;210354;57280;229777;17284;199135;62422;241031;29069;203720;49579;219040;4480;197112;66037;256896;42398;212398;58821;232334;20358;200153;63452;244101;32144;205250;51632;221596;7553;197618;65001;250754;37270;208312;55226;226709;14211;198629;61392;237961;25994;202190;47527;216996;1408;197118]  distributed_mem=Block RAM  rst=off  init_reg=0  en=off  latency=1  arith_type=Unsigned  n_bits=18  bin_pt=0  dbl_ovrd=off  optimize=Area  use_rpm=on  block_type=sprom
      settings: AttributesFormatString=depth = %<depth>\ndist_mem = %<distributed_mem>  xl_area=[0 0 1 0 0 0 0]  block_version=10.1.3
  w : Outport  OutDataType=sfix(16)  OutScaling=2^0
  wires:
  mem_c/1 -> w/1
  addr_sel/1 -> mem_c/1
  Counter/1 -> addr_sel/1
  sync_in/1 -> Counter/1

== system pfb_fft/r4_dit_fft/r4_dit_stage_5/r4_twiddle/twiddle_gen3 ==
  sync_in : Inport  OutDataType=sfix(16)  OutScaling=2^0
  Counter : xbsIndex_r4/Counter  cnt_type=Free Running  cnt_to=Inf  operation=Up  start_count=0  cnt_by_val=1  arith_type=Unsigned  n_bits=8  bin_pt=0  load_pin=off  rst=on  en=off  explicit_period=off  period=1  dbl_ovrd=off  use_behavioral_HDL=off  use_rpm=on  implementation=Fabric  block_type=counter
      settings: xl_area=[4 8 0 8 0 0 0]
  addr_sel : xbsIndex_r4/Slice  nbits=8  boolean_output=off  mode=Upper Bit Location + Width  bit1=0  base1=MSB of Input  bit0=-1  base0=MSB of Input  dbl_ovrd=off  block_type=slice
      settings: infoedit="Extracts a given range of bits from each input sample and presents it at the output.  The output type is ordinarily unsigned with binary point at zero, but can be Boolean when the slice is one bit wide.<P><P>Hardware notes: In hardware this block costs nothing."  block_version=10.1.3
  mem_c : xbsIndex_r4/ROM  depth=256  initVector=[65536;215973;25482;201777;54713;198119;249730;225898;62939;204740;7041;211537;41885;197133;231823;243322;65517;209844;16260;205890;49066;197114;240519;234100;59849;200661;259456;218207;34194;198687;223641;252543;66039;212908;20870;203834;52145;197616;245125;229999;61394;202700;1920;214616;38295;197654;227732;247933;64484;207292;11650;208458;45475;196611;235915;238711;57281;199646;254337;221797;30094;199720;219551;257664;66043;214441;23432;202805;53685;198124;247171;227949;62422;203720;4480;213077;40346;197137;229777;245372;65001;208312;14211;207430;47527;197118;237961;236662;58821;200153;256896;220258;32144;199204;221596;255103;65522;211376;18821;204862;50606;197109;242566;232050;60878;201680;261504;216668;36245;198171;225686;250494;63967;205760;9089;209998;43936;196616;233869;240761;56253;198626;252290;223848;27532;200749;218018;259712;66046;215463;24457;202291;54199;198121;248707;226924;62937;204230;5504;212563;40860;197135;230800;244347;65003;209334;15235;206404;48040;197116;239496;235125;59335;200663;257920;219232;33169;198689;222619;254079;65524;212398;19846;204348;51119;197619;244101;231025;61392;202190;896;215642;37270;197656;226709;248957;63970;206782;10626;209484;44962;196613;234892;239736;56767;199136;253313;222822;28557;200234;219041;258688;66041;213931;21895;203319;52659;197614;246148;228974;61908;203210;2944;214103;39321;197652;228755;246908;64486;207802;12674;207944;46501;196609;236938;237687;58307;199644;255873;220771;31119;199718;220574;256127;65520;210866;17284;205376;49580;197111;241543;233075;60363;201171;260480;217181;35219;198173;224664;251518;63453;205250;8065;211023;42911;196618;232846;242298;55739;198629;250754;224873;26507;201263;216996;261248]  distributed_mem=Block RAM  rst=off  init_reg=0  en=off  latency=1  arith_type=Unsigned  n_bits=18  bin_pt=0  dbl_ovrd=off  optimize=Area  use_rpm=on  block_type=sprom
      settings: AttributesFormatString=depth = %<depth>\ndist_mem = %<distributed_mem>  xl_area=[0 0 1 0 0 0 0]  block_version=10.1.3
  w : Outport  OutDataType=sfix(16)  OutScaling=2^0
  wires:
  mem_c/1 -> w/1
  addr_sel/1 -> mem_c/1
  Counter/1 -> addr_sel/1
  sync_in/1 -> Counter/1

== system pfb_fft/r4_dit_fft/r4_dit_stage_1/quadplex_commutator/biplex_commutator_01/delay_b ==
  in : Inport  OutDataType=sfix(16)  OutScaling=2^0
  Constant : xbsIndex_r4/Constant  arith_type=Boolean  const=1  n_bits=1  bin_pt=0  explicit_period=on  period=1  equ=P=C  opselect=C  inp2=PCIN>>17  opr=+  inp1=P  carry=CIN  dbl_ovrd=off  block_type=constant
  Counter : xbsIndex_r4/Counter  cnt_type=Count Limited  cnt_to=254  operation=Up  start_count=0  cnt_by_val=1  arith_type=Unsigned  n_bits=8  bin_pt=0  load_pin=off  rst=off  en=off  explicit_period=off  period=1  dbl_ovrd=off  use_behavioral_HDL=off  use_rpm=on  implementation=Fabric  block_type=counter
      settings: xl_area=[6 8 0 11 0 0 0]
  bram : xbsIndex_r4/Single Port RAM  depth=256  initVector=0  distributed_mem=Block RAM  write_mode=Read Before Write  rst=off  init_reg=0  en=off  latency=1  dbl_ovrd=off  optimize=Area  use_rpm=off  block_type=spram
      settings: xl_area=[0 0 1 0 0 0 0]  block_version=10.1.3
  out : Outport  OutDataType=sfix(16)  OutScaling=2^0
  wires:
  Constant/1 -> bram/3
  in/1 -> bram/2
  bram/1 -> out/1
  Counter/1 -> bram/1

== system pfb_fft/r4_dit_fft/r4_dit_stage_1/quadplex_commutator/biplex_commutator_01/delay_lo ==
  in : Inport  OutDataType=sfix(16)  OutScaling=2^0
  Constant : xbsIndex_r4/Constant  arith_type=Boolean  const=1  n_bits=1  bin_pt=0  explicit_period=on  period=1  equ=P=C  opselect=C  inp2=PCIN>>17  opr=+  inp1=P  carry=CIN  dbl_ovrd=off  block_type=constant
  Counter : xbsIndex_r4/Counter  cnt_type=Count Limited  cnt_to=254  operation=Up  start_count=0  cnt_by_val=1  arith_type=Unsigned  n_bits=8  bin_pt=0  load_pin=off  rst=off  en=off  explicit_period=off  period=1  dbl_ovrd=off  use_behavioral_HDL=off  use_rpm=on  implementation=Fabric  block_type=counter
      settings: xl_area=[6 8 0 11 0 0 0]
  bram : xbsIndex_r4/Single Port RAM  depth=256  initVector=0  distributed_mem=Block RAM  write_mode=Read Before Write  rst=off  init_reg=0  en=off  latency=1  dbl_ovrd=off  optimize=Area  use_rpm=off  block_type=spram
      settings: xl_area=[0 0 1 0 0 0 0]  block_version=10.1.3
  out : Outport  OutDataType=sfix(16)  OutScaling=2^0
  wires:
  Constant/1 -> bram/3
  in/1 -> bram/2
  bram/1 -> out/1
  Counter/1 -> bram/1

== system pfb_fft/r4_dit_fft/r4_dit_stage_1/quadplex_commutator/biplex_commutator_23/delay_b ==
  in : Inport  OutDataType=sfix(16)  OutScaling=2^0
  Constant : xbsIndex_r4/Constant  arith_type=Boolean  const=1  n_bits=1  bin_pt=0  explicit_period=on  period=1  equ=P=C  opselect=C  inp2=PCIN>>17  opr=+  inp1=P  carry=CIN  dbl_ovrd=off  block_type=constant
  Counter : xbsIndex_r4/Counter  cnt_type=Count Limited  cnt_to=254  operation=Up  start_count=0  cnt_by_val=1  arith_type=Unsigned  n_bits=8  bin_pt=0  load_pin=off  rst=off  en=off  explicit_period=off  period=1  dbl_ovrd=off  use_behavioral_HDL=off  use_rpm=on  implementation=Fabric  block_type=counter
      settings: xl_area=[6 8 0 11 0 0 0]
  bram : xbsIndex_r4/Single Port RAM  depth=256  initVector=0  distributed_mem=Block RAM  write_mode=Read Before Write  rst=off  init_reg=0  en=off  latency=1  dbl_ovrd=off  optimize=Area  use_rpm=off  block_type=spram
      settings: xl_area=[0 0 1 0 0 0 0]  block_version=10.1.3
  out : Outport  OutDataType=sfix(16)  OutScaling=2^0
  wires:
  Constant/1 -> bram/3
  in/1 -> bram/2
  bram/1 -> out/1
  Counter/1 -> bram/1

== system pfb_fft/r4_dit_fft/r4_dit_stage_1/quadplex_commutator/biplex_commutator_23/delay_lo ==
  in : Inport  OutDataType=sfix(16)  OutScaling=2^0
  Constant : xbsIndex_r4/Constant  arith_type=Boolean  const=1  n_bits=1  bin_pt=0  explicit_period=on  period=1  equ=P=C  opselect=C  inp2=PCIN>>17  opr=+  inp1=P  carry=CIN  dbl_ovrd=off  block_type=constant
  Counter : xbsIndex_r4/Counter  cnt_type=Count Limited  cnt_to=254  operation=Up  start_count=0  cnt_by_val=1  arith_type=Unsigned  n_bits=8  bin_pt=0  load_pin=off  rst=off  en=off  explicit_period=off  period=1  dbl_ovrd=off  use_behavioral_HDL=off  use_rpm=on  implementation=Fabric  block_type=counter
      settings: xl_area=[6 8 0 11 0 0 0]
  bram : xbsIndex_r4/Single Port RAM  depth=256  initVector=0  distributed_mem=Block RAM  write_mode=Read Before Write  rst=off  init_reg=0  en=off  latency=1  dbl_ovrd=off  optimize=Area  use_rpm=off  block_type=spram
      settings: xl_area=[0 0 1 0 0 0 0]  block_version=10.1.3
  out : Outport  OutDataType=sfix(16)  OutScaling=2^0
  wires:
  Constant/1 -> bram/3
  in/1 -> bram/2
  bram/1 -> out/1
  Counter/1 -> bram/1

== system pfb_fft/r4_dit_fft/r4_dit_stage_1/quadplex_commutator/biplex_commutator_ac/delay_b ==
  in : Inport  OutDataType=sfix(16)  OutScaling=2^0
  Constant : xbsIndex_r4/Constant  arith_type=Boolean  const=1  n_bits=1  bin_pt=0  explicit_period=on  period=1  equ=P=C  opselect=C  inp2=PCIN>>17  opr=+  inp1=P  carry=CIN  dbl_ovrd=off  block_type=constant
  Counter : xbsIndex_r4/Counter  cnt_type=Count Limited  cnt_to=510  operation=Up  start_count=0  cnt_by_val=1  arith_type=Unsigned  n_bits=9  bin_pt=0  load_pin=off  rst=off  en=off  explicit_period=off  period=1  dbl_ovrd=off  use_behavioral_HDL=off  use_rpm=on  implementation=Fabric  block_type=counter
      settings: xl_area=[7 9 0 12 0 0 0]
  bram : xbsIndex_r4/Single Port RAM  depth=512  initVector=0  distributed_mem=Block RAM  write_mode=Read Before Write  rst=off  init_reg=0  en=off  latency=1  dbl_ovrd=off  optimize=Area  use_rpm=off  block_type=spram
      settings: xl_area=[0 0 1 0 0 0 0]  block_version=10.1.3
  out : Outport  OutDataType=sfix(16)  OutScaling=2^0
  wires:
  Constant/1 -> bram/3
  in/1 -> bram/2
  bram/1 -> out/1
  Counter/1 -> bram/1
